simulink model "Model_V3_vertical"  (R2024a)
settings: Solver=ode4  StartTime=0.0  StopTime=15  FixedStep=0.0001  RelTol=1e-3
values from neighbouring files (symbols this model uses):
  C = b0    (= 1.4)    [rodas_v2.m]    (also in varglobal.m = 4000)
  Kf = 13000    [varglobal.m]
  Kp = 200000    [varglobal.m]
  re = 0.3    [varglobal.m]
undefined symbols (not defined in the file or in its folder): eqmovimento, rodas, Transformador, TransformadorT
libraries: simulink_extras x1
settings Model: Creator=Vilson Wenis Belle  LastModifiedBy=wenis
settings SolverCC: AlgebraicLoopSolver=TrustRegion
settings DebuggingCC: UnconnectedInputMsg=warning  UnconnectedOutputMsg=warning  UnconnectedLineMsg=warning
settings ModelReferenceCC: EnableRefExpFcnMdlSchedulingChecks=on
settings RTWCC: GPUComputeCapability=3.5  DLArmComputeVersion=19.05

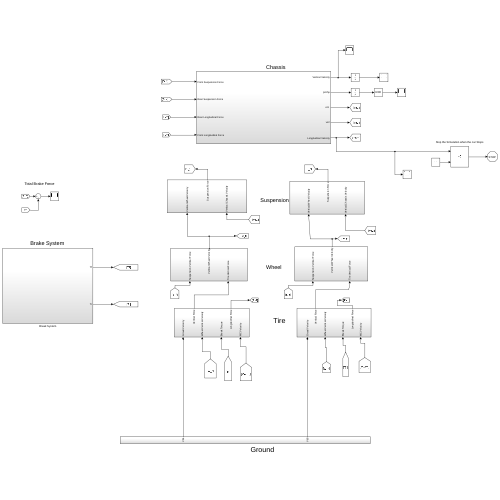
[thumbnail: Simulink's stored preview of the top-level diagram]
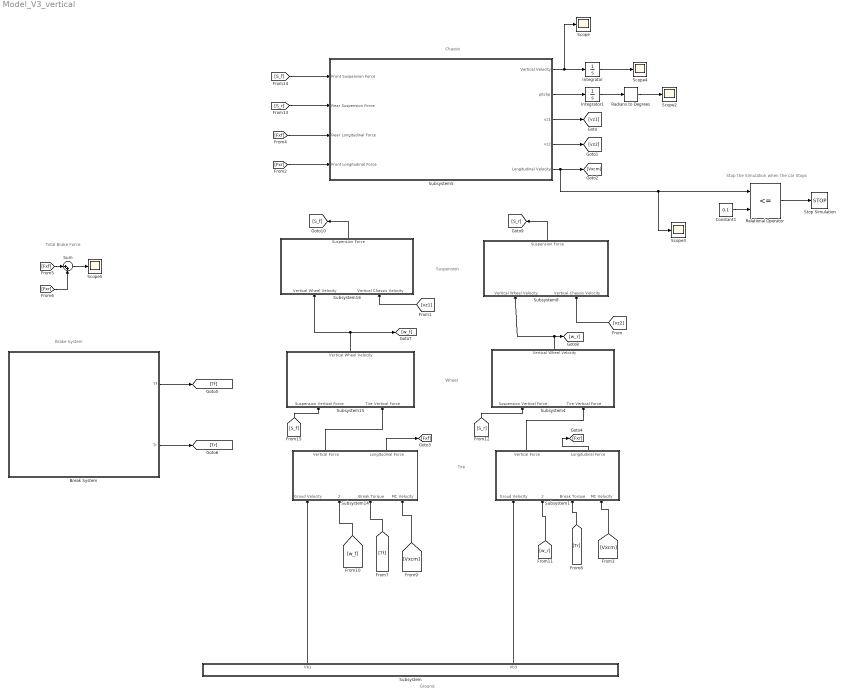
== system Model_V3_vertical ==
  note: Stop the Simulation when the car Stops
  note: Chassis
  note: Suspension
  note: Wheel
  note: Total Brake Force
  note: Brake System
  note: Ground
  note: Tire
  Break System : Subsystem
  Constant1 : Constant  Value=0.1
  Integrator : Integrator
  Integrator1 : Integrator
  Radians to Degrees : simulink_extras/Transformations/Radians to Degrees
  Relational Operator : RelationalOperator  Operator=<=  OutDataTypeStr=boolean  RndMeth=Simplest  InputSameDT=off
  Scope{,2..5} (5 alike) : Scope
  Stop Simulation : Stop
  Subsystem : Subsystem
  Subsystem1 : Subsystem
  Subsystem14 : Subsystem
  Subsystem15 : Subsystem
  Subsystem16 : Subsystem
  Subsystem4 : Subsystem
  Subsystem5 : Subsystem
  Subsystem8 : Subsystem
  Sum : Sum  Inputs=|++
  wires:
  Subsystem15/1(Vertical Wheel Velocity) -> [w_f], Subsystem16/1(Vertical Wheel Velocity)
  Subsystem14/1(Vertical Force) -> Subsystem15/2(Tire Vertical Force)
  Subsystem5/1(Vertical Velocity) -> Integrator/1, Scope/1
  Integrator/1 -> Scope4/1
  Subsystem/2(Vb3) -> Subsystem1/1(Groud Velocity)
  Integrator1/1 -> Radians to Degrees/1
  Subsystem5/2(pitchp) -> Integrator1/1
  Radians to Degrees/1 -> Scope2/1
  Subsystem/1(Vb1) -> Subsystem14/1(Groud Velocity)
  Subsystem5/3("vz1 ") -> [vz1]
  Subsystem5/4(vz2) -> [vz2]
  [vz2] -> Subsystem8/2(Vertical Chassis Velocity)
  [vz1] -> Subsystem16/2(Vertical Chassis Velocity)
  [Vxcm] -> Subsystem1/4(MC Velocity)
  Subsystem14/2(Longitudinal Force) -> [Fxf]
  [Fxf] -> Subsystem5/3(Rear Longitudinal Force)
  Subsystem1/2(Longitudinal Force) -> [Fxr]
  [Fxr] -> Subsystem5/4(Front Longitudinal Force)
  Relational Operator/1 -> Stop Simulation/1
  Subsystem5/5(Longitudinal Velocity) -> [Vxcm], Relational Operator/1, Scope3/1
  Constant1/1 -> Relational Operator/2
  [Fxf] -> Sum/1
  [Fxr] -> Sum/2
  Sum/1 -> Scope5/1
  Break System/1(Tf) -> [Tf]
  [Tf] -> Subsystem14/3(Break Torque)
  Break System/2(Tr) -> [Tr]
  [Tr] -> Subsystem1/3(Break Torque)
  [Vxcm] -> Subsystem14/4(MC Velocity)
  Subsystem4/1(Vertical Wheel Velocity) -> Subsystem8/1(Vertical Wheel Velocity), [w_r]
  Subsystem1/1(Vertical Force) -> Subsystem4/2(Tire Vertical Force)
  [w_f] -> Subsystem14/2(Wheel Vertical Velocity)
  [w_r] -> Subsystem1/2(Wheel Vertical Velocity)
  Subsystem8/1(Suspension Force) -> [S_r]
  [S_r] -> Subsystem4/1(Suspension Vertical Force)
  [S_r] -> Subsystem5/2(Rear Suspension Force)
  [S_f] -> Subsystem5/1(Front Suspension Force)
  Subsystem16/1(Suspension Force) -> [S_f]
  [S_f] -> Subsystem15/1(Suspension Vertical Force)

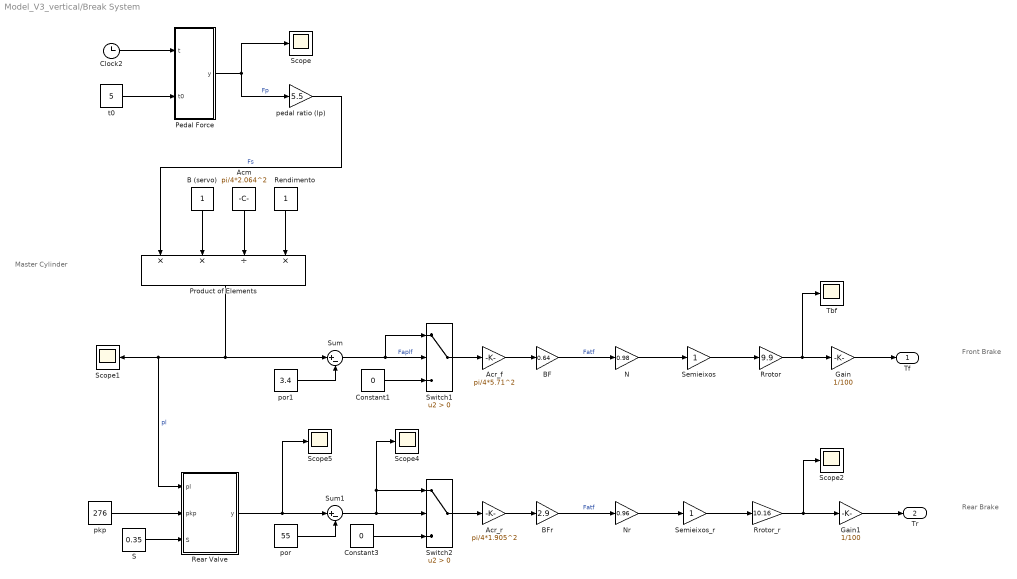
== system Model_V3_vertical/Break System ==
  note: Master Cylinder
  note: Front Brake
  note: Rear Brake
  Acm : Constant  Value=pi/4*2.064^2
  Acr_f : Gain  Gain=pi/4*5.71^2
  Acr_r : Gain  Gain=pi/4*1.905^2
  B (servo) : Constant
  BF : Gain  Gain=0.64
  BFr : Gain  Gain=2.9
  Clock2 : Clock
  Constant1 : Constant  Value=0
  Constant3 : Constant  Value=0
  Gain : Gain  Gain=1/100
  Gain1 : Gain  Gain=1/100
  N : Gain  Gain=0.98
  Nr : Gain  Gain=0.96
  Pedal Force : MATLAB Function  TreatAsAtomicUnit=on
  Product of Elements : Product  Inputs=**/*
  Rear Valve : MATLAB Function  TreatAsAtomicUnit=on
  Rendimento : Constant
  Rrotor : Gain  Gain=9.9
  Rrotor_r : Gain  Gain=10.16
  S : Constant  Value=0.35
  Scope{,1..2,4..5} (5 alike) : Scope
  Semieixos : Gain
  Semieixos_r : Gain
  Sum : Sum  Inputs=|+-
  Sum1 : Sum  Inputs=|+-
  Switch1 : Switch  Criteria=u2 > Threshold  SaturateOnIntegerOverflow=off  InputSameDT=off
  Switch2 : Switch  Criteria=u2 > Threshold  SaturateOnIntegerOverflow=off  InputSameDT=off
  Tbf : Scope
  pedal ratio (lp) : Gain  Gain=5.5
  pkp : Constant  Value=276
  por : Constant  Value=55
  por1 : Constant  Value=3.4
  t0 : Constant  Value=5
  Tf : Outport
  Tr : Outport  Port=2
  wires:
  Acm/1 -> Product of Elements/3
  Semieixos/1 -> Rrotor/1
  Switch1/1 -> Acr_f/1
  Rendimento/1 -> Product of Elements/4
  Switch2/1 -> Acr_r/1
  Clock2/1 -> Pedal Force/1(t)
  por1/1 -> Sum/2
  Rear Valve/1(y) -> Sum1/1, Scope5/1
  N/1 -> Semieixos/1
  BF/1 -> N/1  "Fatf"
  S/1 -> Rear Valve/3(S)
  Pedal Force/1(y) -> Scope/1, pedal ratio (lp)/1  "Fp"
  Acr_f/1 -> BF/1
  Constant1/1 -> Switch1/3
  Sum/1 -> Switch1/1, Switch1/2  "Faplf"
  pkp/1 -> Rear Valve/2(pkp)
  Product of Elements/1 -> Scope1/1, Rear Valve/1(pl), Sum/1  "pl"
  Rrotor/1 -> Gain/1, Tbf/1
  B (servo)/1 -> Product of Elements/2
  Semieixos_r/1 -> Rrotor_r/1
  BFr/1 -> Nr/1  "Fatf"
  t0/1 -> Pedal Force/2(t0)
  Acr_r/1 -> BFr/1
  Nr/1 -> Semieixos_r/1
  pedal ratio (lp)/1 -> Product of Elements/1  "Fs"
  Sum1/1 -> Switch2/2, Switch2/1, Scope4/1
  por/1 -> Sum1/2
  Constant3/1 -> Switch2/3
  Rrotor_r/1 -> Gain1/1, Scope2/1
  Gain/1 -> Tf/1
  Gain1/1 -> Tr/1

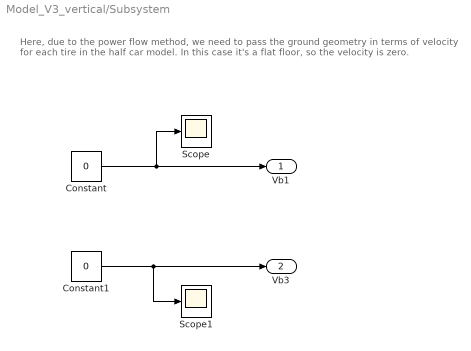
== system Model_V3_vertical/Subsystem ==
  note: Here, due to the power flow method, we need to pass the ground geometry in terms of velocity for each tire in the half car model. In this case it's a flat floor, so the velocity is zero.
  Constant : Constant  Value=0
  Constant1 : Constant  Value=0
  Scope : Scope
  Scope1 : Scope
  Vb1 : Outport
  Vb3 : Outport  Port=2
  wires:
  Constant/1 -> Scope/1, Vb1/1
  Constant1/1 -> Scope1/1, Vb3/1

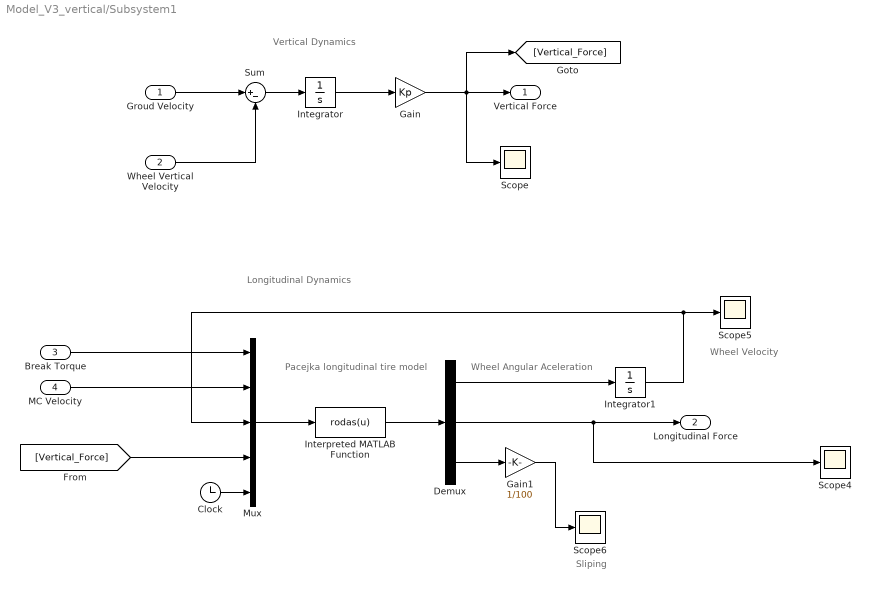
== system Model_V3_vertical/Subsystem1 ==
  note: Wheel Velocity
  note: Pacejka longitudinal tire model
  note: Vertical Dynamics
  note: Longitudinal Dynamics
  note: Wheel Angular Aceleration
  note: Sliping
  Groud Velocity : Inport
  Wheel Vertical Velocity : Inport  Port=2
  Break Torque : Inport  Port=3
  MC Velocity : Inport  Port=4
  Clock : Clock
  Demux : Demux  Outputs=3
  Gain : Gain  Gain=Kp
  Gain1 : Gain  Gain=1/100
  Integrator : Integrator  InitialCondition=-0.003
  Integrator1 : Integrator  InitialCondition=30/re  LimitOutput=on  LowerSaturationLimit=0
  Interpreted MATLAB Function : MATLABFcn  MATLABFcn=rodas(u)  OutputDimensions=3
  Mux : Mux  Inputs=5
  Scope{,4..6} (4 alike) : Scope
  Sum : Sum  Inputs=|+-
  Vertical Force : Outport
  Longitudinal Force : Outport  Port=2
  wires:
  Integrator/1 -> Gain/1
  Demux/1 -> Integrator1/1
  Sum/1 -> Integrator/1
  Interpreted MATLAB Function/1 -> Demux/1
  Wheel Vertical Velocity/1 -> Sum/2
  Clock/1 -> Mux/5
  Gain1/1 -> Scope6/1
  Gain/1 -> Scope/1, [Vertical_Force], Vertical Force/1
  Mux/1 -> Interpreted MATLAB Function/1
  Demux/3 -> Gain1/1
  Groud Velocity/1 -> Sum/1
  Break Torque/1 -> Mux/1
  MC Velocity/1 -> Mux/2
  [Vertical_Force] -> Mux/4
  Integrator1/1 -> Mux/3, Scope5/1
  Demux/2 -> Scope4/1, Longitudinal Force/1

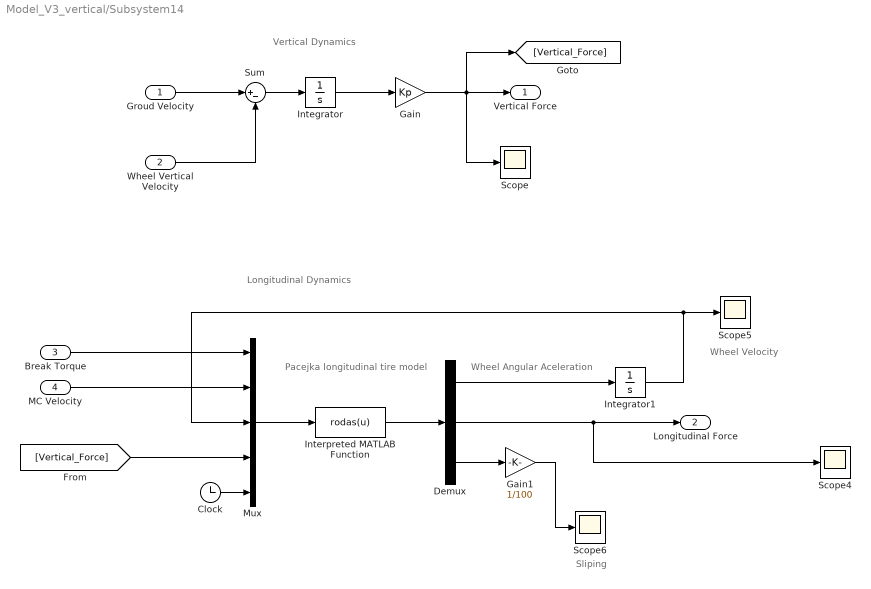
== system Model_V3_vertical/Subsystem14 ==
  note: Wheel Velocity
  note: Sliping
  note: Wheel Angular Aceleration
  note: Longitudinal Dynamics
  note: Pacejka longitudinal tire model
  note: Vertical Dynamics
  Groud Velocity : Inport
  Wheel Vertical Velocity : Inport  Port=2
  Break Torque : Inport  Port=3
  MC Velocity : Inport  Port=4
  Clock : Clock
  Demux : Demux  Outputs=3
  Gain : Gain  Gain=Kp
  Gain1 : Gain  Gain=1/100
  Integrator : Integrator  InitialCondition=-0.003
  Integrator1 : Integrator  InitialCondition=30/re  LimitOutput=on  LowerSaturationLimit=0
  Interpreted MATLAB Function : MATLABFcn  MATLABFcn=rodas(u)  OutputDimensions=3
  Mux : Mux  Inputs=5
  Scope{,4..6} (4 alike) : Scope
  Sum : Sum  Inputs=|+-
  Vertical Force : Outport
  Longitudinal Force : Outport  Port=2
  wires:
  Wheel Vertical Velocity/1 -> Sum/2
  Groud Velocity/1 -> Sum/1
  Sum/1 -> Integrator/1
  Integrator/1 -> Gain/1
  Gain/1 -> Scope/1, [Vertical_Force], Vertical Force/1
  Break Torque/1 -> Mux/1
  Mux/1 -> Interpreted MATLAB Function/1
  Demux/1 -> Integrator1/1
  Demux/2 -> Scope4/1, Longitudinal Force/1
  Interpreted MATLAB Function/1 -> Demux/1
  Demux/3 -> Gain1/1
  Gain1/1 -> Scope6/1
  MC Velocity/1 -> Mux/2
  Integrator1/1 -> Mux/3, Scope5/1
  Clock/1 -> Mux/5
  [Vertical_Force] -> Mux/4

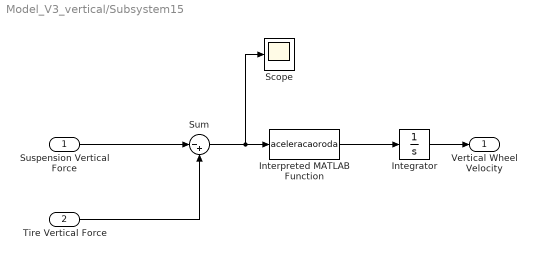
== system Model_V3_vertical/Subsystem15 ==
  Suspension Vertical Force : Inport
  Tire Vertical Force : Inport  Port=2
  Integrator : Integrator
  Interpreted MATLAB Function : MATLABFcn  MATLABFcn=aceleracaoroda  OutputDimensions=1
  Scope : Scope
  Sum : Sum  Inputs=|-+
  Vertical Wheel Velocity : Outport
  wires:
  Suspension Vertical Force/1 -> Sum/1
  Tire Vertical Force/1 -> Sum/2
  Integrator/1 -> Vertical Wheel Velocity/1
  Sum/1 -> Scope/1, Interpreted MATLAB Function/1
  Interpreted MATLAB Function/1 -> Integrator/1

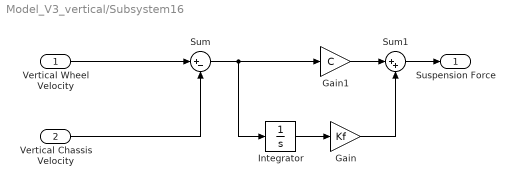
== system Model_V3_vertical/Subsystem16 ==
  Vertical Wheel Velocity : Inport
  Vertical Chassis Velocity : Inport  Port=2
  Gain : Gain  Gain=Kf
  Gain1 : Gain  Gain=C
  Integrator : Integrator
  Sum : Sum  Inputs=|+-
  Sum1 : Sum  Inputs=|++
  Suspension Force : Outport
  wires:
  Vertical Chassis Velocity/1 -> Sum/2
  Vertical Wheel Velocity/1 -> Sum/1
  Sum/1 -> Gain1/1, Integrator/1
  Integrator/1 -> Gain/1
  Gain1/1 -> Sum1/1
  Gain/1 -> Sum1/2
  Sum1/1 -> Suspension Force/1

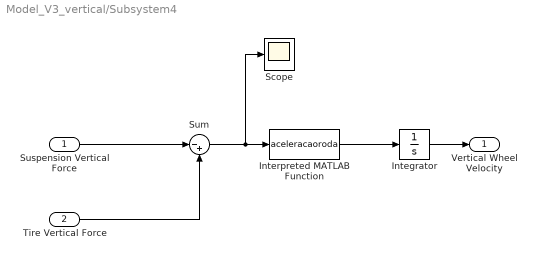
== system Model_V3_vertical/Subsystem4 ==
  Suspension Vertical Force : Inport
  Tire Vertical Force : Inport  Port=2
  Integrator : Integrator
  Interpreted MATLAB Function : MATLABFcn  MATLABFcn=aceleracaoroda  OutputDimensions=1
  Scope : Scope
  Sum : Sum  Inputs=|-+
  Vertical Wheel Velocity : Outport
  wires:
  Integrator/1 -> Vertical Wheel Velocity/1
  Sum/1 -> Scope/1, Interpreted MATLAB Function/1
  Interpreted MATLAB Function/1 -> Integrator/1
  Tire Vertical Force/1 -> Sum/2
  Suspension Vertical Force/1 -> Sum/1

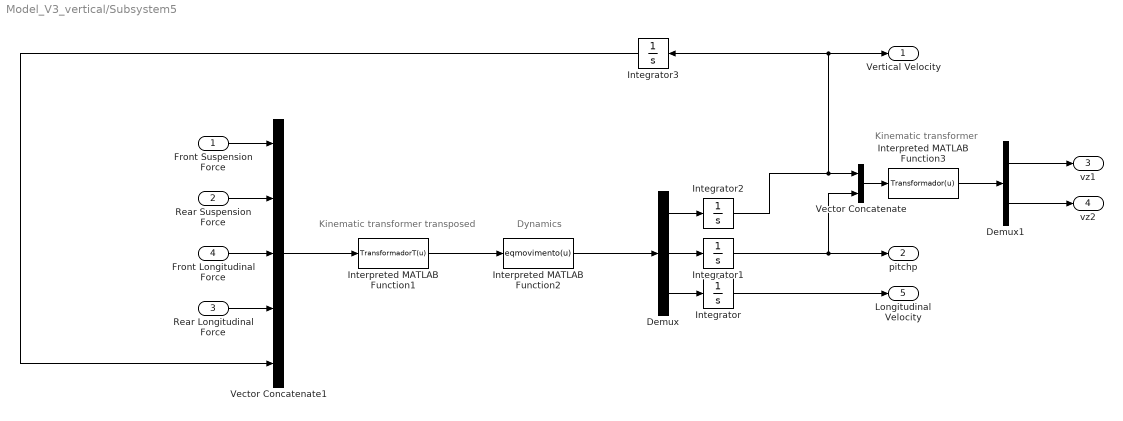
== system Model_V3_vertical/Subsystem5 ==
  note: Kinematic transformer transposed
  note: Dynamics
  note: Kinematic transformer
  Front Suspension Force : Inport
  Rear Suspension Force : Inport  Port=2
  Rear Longitudinal Force : Inport  Port=3
  Front Longitudinal Force : Inport  Port=4
  Demux : Demux  Outputs=3
  Demux1 : Demux  Outputs=2
  Integrator : Integrator  InitialCondition=30
  Integrator1 : Integrator
  Integrator2 : Integrator
  Integrator3 : Integrator
  Interpreted MATLAB Function1 : MATLABFcn  MATLABFcn=TransformadorT(u)  OutputDimensions=3
  Interpreted MATLAB Function2 : MATLABFcn  MATLABFcn=eqmovimento(u)  OutputDimensions=3
  Interpreted MATLAB Function3 : MATLABFcn  MATLABFcn=Transformador(u)  OutputDimensions=2
  Vector Concatenate : Concatenate
  Vector Concatenate1 : Concatenate  NumInputs=5
  Vertical Velocity : Outport
  pitchp : Outport  Port=2
  "vz1 " : Outport  Port=3
  vz2 : Outport  Port=4
  Longitudinal Velocity : Outport  Port=5
  wires:
  Demux1/2 -> vz2/1
  Demux1/1 -> "vz1 "/1
  Vector Concatenate1/1 -> Interpreted MATLAB Function1/1
  Rear Suspension Force/1 -> Vector Concatenate1/2
  Front Suspension Force/1 -> Vector Concatenate1/1
  Interpreted MATLAB Function2/1 -> Demux/1
  Demux/1 -> Integrator2/1
  Demux/2 -> Integrator1/1
  Integrator2/1 -> Vertical Velocity/1, Integrator3/1, Vector Concatenate/1
  Vector Concatenate/1 -> Interpreted MATLAB Function3/1
  Integrator1/1 -> Vector Concatenate/2, pitchp/1
  Interpreted MATLAB Function3/1 -> Demux1/1
  Rear Longitudinal Force/1 -> Vector Concatenate1/4
  Front Longitudinal Force/1 -> Vector Concatenate1/3
  Integrator3/1 -> Vector Concatenate1/5
  Interpreted MATLAB Function1/1 -> Interpreted MATLAB Function2/1
  Integrator/1 -> Longitudinal Velocity/1
  Demux/3 -> Integrator/1

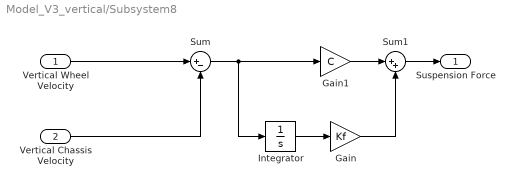
== system Model_V3_vertical/Subsystem8 ==
  Vertical Wheel Velocity : Inport
  Vertical Chassis Velocity : Inport  Port=2
  Gain : Gain  Gain=Kf
  Gain1 : Gain  Gain=C
  Integrator : Integrator
  Sum : Sum  Inputs=|+-
  Sum1 : Sum  Inputs=|++
  Suspension Force : Outport
  wires:
  Sum/1 -> Gain1/1, Integrator/1
  Gain1/1 -> Sum1/1
  Vertical Chassis Velocity/1 -> Sum/2
  Integrator/1 -> Gain/1
  Sum1/1 -> Suspension Force/1
  Gain/1 -> Sum1/2
  Vertical Wheel Velocity/1 -> Sum/1

== matlab function Model_V3_vertical/Break System/Rear Valve ==
  data: pl input; y output; pkp input; S input
function y = fcn(pl, pkp, S)



if pl <= pkp
    y = pl;
else
    y = pkp + S*(pl-pkp);
end

end

== matlab function Model_V3_vertical/Break System/Pedal Force ==
  data: t input; y output; t0 input
function y = fcn(t, t0)


if t<=t0
    y=0;
else
    y = 700;
end
